simulink model "boost_fixed_irradiance"  (R2024b)
settings: Solver=ode5  StartTime=0.0  StopTime=5  MaxStep=1e-3  RelTol=1e-3
libraries: spsSeriesRLCBranchLib x3, spsCurrentMeasurementLib x1, spsDiodeLib x1, spsMosfetLib x1, slpidlib x1, spsPVArrayLib x1, spsPWMGeneratorDCDCLib x1, simulink x1, spsVoltageMeasurementLib x1, spspowerguiLib x1
settings Model: Creator=30698  LastModifiedBy=strat
settings SolverCC: AlgebraicLoopSolver=TrustRegion
settings DebuggingCC: UnconnectedInputMsg=warning  UnconnectedOutputMsg=warning  UnconnectedLineMsg=warning
settings ModelReferenceCC: EnableRefExpFcnMdlSchedulingChecks=on
settings RTWCC: GPUComputeCapability=3.5  DLArmComputeVersion=19.05

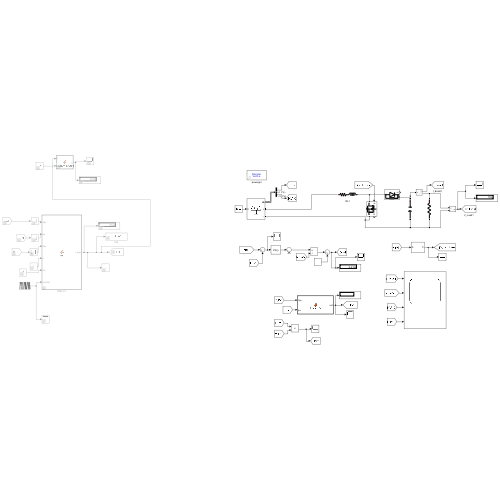
[thumbnail: Simulink's stored preview of the top-level diagram]
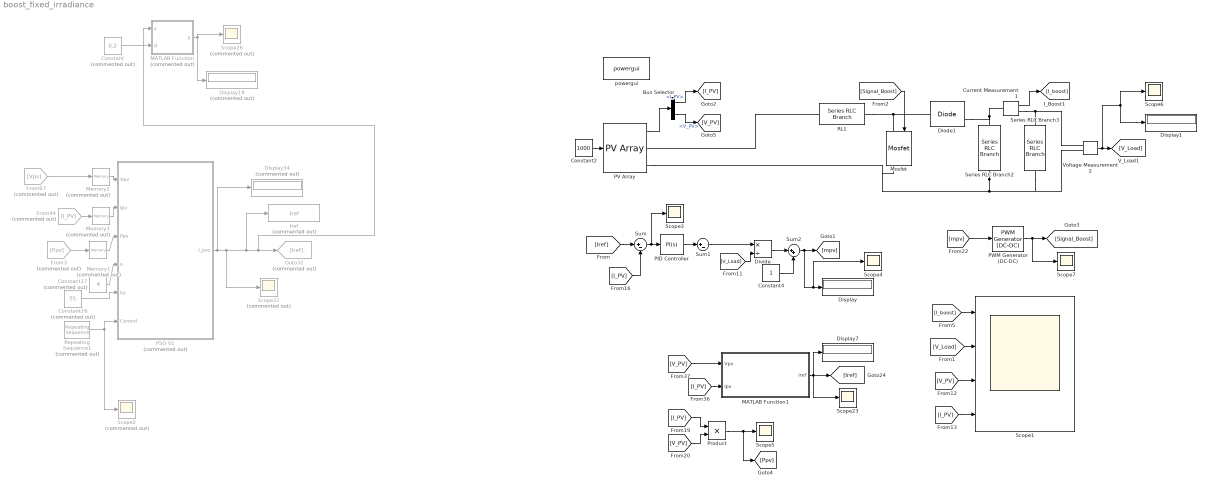
== system boost_fixed_irradiance ==
  Bus Selector : BusSelector  OutputSignals=I_PV,V_PV
  Constant : Constant  Commented=on  Value=0.2
  Constant16 : Constant  Commented=on  Value=55
  Constant17 : Constant  Commented=on  Value=4
  Constant2 : Constant  Value=1000
  Constant4 : Constant
  Current Measurement1 : spsCurrentMeasurementLib/Current Measurement  PhasorSimulation=off  OutputType=Complex  PSBequivalent=0
  Diode1 : spsDiodeLib/Diode  Ron=0.001  Lon=0  Vf=0.8  IC=0  UseSnubber=0  Rs=500  Cs=250e-9  Measurements=on
  Display : Display
  Display1 : Display
  Display19 : Display  Commented=on
  Display34 : Display  Commented=on
  Display7 : Display
  Divide : Product  Inputs=*/
  From3 : From  Commented=on  GotoTag=Ppv
  From44 : From  Commented=on  GotoTag=I_PV
  From67 : From  Commented=on  GotoTag=Vpv
  Goto32 : Goto  Commented=on  GotoTag=Iref
  Iref : ToWorkspace  Commented=on  VariableName=Iref  SaveFormat=Timeseries  SampleTime=-1
  MATLAB Function : MATLAB Function  Commented=on  TreatAsAtomicUnit=on
  MATLAB Function1 : MATLAB Function  TreatAsAtomicUnit=on
  Memory1 : Memory  Commented=on  InheritSampleTime=on
  Memory2 : Memory  Commented=on  InheritSampleTime=on
  Memory3 : Memory  Commented=on  InheritSampleTime=on
  Mosfet : spsMosfetLib/Mosfet  Ron=0.1  Lon=0  Rd=0.01  Vfd=0  IC=0  Rs=1e5  Cs=inf  Measurements=on
  PID Controller : slpidlib/PID Controller  Controller=PI  Form=Parallel  TimeDomain=Continuous-time  UseExternalTs=off  SampleTime=-1  IntegratorMethod=Forward Euler  FilterMethod=Forward Euler  ControllerParametersSource=internal  P=15  I=100  UseKiTs=off  D=0  UseExternalDerivativeSource=off  N=100  UseFilter=on  TunerSelectOption=Frequency Response Based  InitialConditionSource=internal  InitialConditionForIntegrator=0  InitialConditionForFilter=0  DifferentiatorICPrevScaledInput=0  ExternalReset=none  TrackingMode=off  Kt=1  LimitOutput=off  SatLimitsSource=internal  UpperSaturationLimit=inf  LowerSaturationLimit=-inf  LinearizeAsGain=on  AntiWindupMode=none  Kb=1  LimitIntegrator=off  UpperIntegratorSaturationLimit=inf  LowerIntegratorSaturationLimit=-inf  POutMin=[]  POutMax=[]  IOutMin=[]  IOutMax=[]  DOutMin=[]  DOutMax=[]  NOutMin=[]  NOutMax=[]  SumOutMin=[]  SumOutMax=[]  SaturationOutMin=[]  SaturationOutMax=[]  PParamMin=[]  PParamMax=[]  IParamMin=[]  IParamMax=[]  DParamMin=[]  DParamMax=[]  NParamMin=[]  NParamMax=[]  KbParamMin=[]  KbParamMax=[]  KtParamMin=[]  KtParamMax=[]  KbOutMin=[]  KbOutMax=[]  KtOutMin=[]  KtOutMax=[]  IntegratorOutMin=[]  IntegratorOutMax=[]  FilterOutMin=[]  FilterOutMax=[]  SumI1OutMin=[]  SumI1OutMax=[]  SumI2OutMin=[]  SumI2OutMax=[]  SumI3OutMin=[]  SumI3OutMax=[]  SumI4OutMin=[]  SumI4OutMax=[]  SumDOutMin=[]  SumDOutMax=[]  DifferentiatorOutMin=[]  DifferentiatorOutMax=[]  FilterDiffOutCoefMin=[]  FilterDiffOutCoefMax=[]  ReciprocalOutMin=[]  ReciprocalOutMax=[]  SumDenOutMin=[]  SumDenOutMax=[]  SumNumOutMin=[]  SumNumOutMax=[]  DivideOutMin=[]  DivideOutMax=[]  UdiffTsProdOutMin=[]  UdiffTsProdOutMax=[]  NTsProdOutMin=[]  NTsProdOutMax=[]  UintegralTsProdOutMin=[]  UintegralTsProdOutMax=[]  UngainTsProdOutMin=[]  UngainTsProdOutMax=[]  ClampingZeroOutDataTypeStr=Inherit: Inherit via back propagation  ClampingZeroOutMin=[]  ClampingZeroOutMax=[]  FilterDenConstantOutDataTypeStr=Inherit: Inherit via back propagation  FilterDenConstantOutMin=[]  FilterDenConstantOutMax=[]  PCopyOutDataTypeStr=Inherit: Inherit via back propagation  PCopyOutMin=[]  PCopyOutMax=[]  NCopyOutDataTypeStr=Inherit: Inherit via back propagation  NCopyOutMin=[]  NCopyOutMax=[]  IntegratorContinuousStateAttributes=''  IntegratorStateMustResolveToSignalObject=off  IntegratorRTWStateStorageClass=Auto  FilterContinuousStateAttributes=''  FilterStateMustResolveToSignalObject=off  FilterRTWStateStorageClass=Auto  ParallelPVariant=InternalParameters  IdealPVariant=Disabled  IVariant=InternalParameters  DVariant=Disabled  IntegratorVariant=Continuous  SatVariant=Disabled  AWVariant=Passthrough  PCopyVariant=Disabled  TRVariant=Disabled  FdbkBlocksVariant=Forward  IdealPFdbkVariant=Disabled  SatFdbkVariant=Disabled  DerivativeFilterVariant=Disabled  NVariant=Disabled  NCopyVariant=Disabled_SignalSpec  FilterICVariant=Disabled  IntegratorICVariant=InternalICs  ExternalResetVariant=Disabled  TRSumVariant=Passthrough  SumFdbkVariant=Disabled  SumVariant=Sum_PI  TsampFilterVariant=InternalTs  TsampNgainVariant=Passthrough  TsampIntegralVariant=Disabled_SignalSpec  ExternalSaturationOutDataTypeStr=Inherit: Same as second input  DerivativeSourceVariant=Disabled  PreIntVariant=InternalPreInt
  PSO V1 : MATLAB Function  Commented=on  TreatAsAtomicUnit=on  SystemSampleTime=1e-2
      settings: MinAlgLoopOccurrences=on
  PV Array : spsPVArrayLib/PV Array  Npar=5  Nser=14.15  PlotType=array @ 1000 W/m2 & specified temperatures  S_vec="[ 1000  500  100 ]"  Temp_C_vec="[ 45 25  ]"  ModuleName=User-defined  PlotWhenSelected=off  Pm=213.15  Ncell=60  Voc=34.7  Isc=7.84  Vm=29  Im=7.35  beta_Voc_pc=-0.36099  alpha_Isc_pc=0.102  beta_Voc=-0.12526  alpha_Isc=0.0079968  IL=7.8455  I0=2.9177e-10  nI=0.938  Rsh=259.7398  Rs=0.18261  RobustModel=on  RobustCellTemperature=25  BAL=on  Tc=1e-6  Tfilter=5e-5
  PWM Generator (DC-DC) : spsPWMGeneratorDCDCLib/PWM Generator (DC-DC)  Fsw=20000  Ts=0
  Product : Product
  RL1 : spsSeriesRLCBranchLib/Series RLC Branch  LConnTagsString=__new0  RConnTagsString=__new0  BranchType=RL  Resistance=0.01  Inductance=8e-3  SetiL0=off  InitialCurrent=0  Capacitance=1e-6  Setx0=off  InitialVoltage=0  Measurements=None
  Repeating Sequence1 : simulink/Sources/Repeating Sequence  Commented=on  rep_seq_t=[0 4.9 5 9 9.9 10 14]  rep_seq_y="[0 1 1 0  1 1 0]"
  Scope1 : Scope  NumInputPorts=4
  Scope2 : Scope  Commented=on
  Scope{3..7,23} (6 alike) : Scope
  Scope26 : Scope  Commented=on
  Scope31 : Scope  Commented=on
  Series RLC Branch2 : spsSeriesRLCBranchLib/Series RLC Branch  LConnTagsString=__new0  RConnTagsString=__new0  BranchType=C  Resistance=1  Inductance=1e-3  SetiL0=off  InitialCurrent=0  Capacitance=1e-2  Setx0=on  InitialVoltage=400  Measurements=None
  Series RLC Branch3 : spsSeriesRLCBranchLib/Series RLC Branch  LConnTagsString=__new0  RConnTagsString=__new0  BranchType=R  Resistance=100  Inductance=1e-3  SetiL0=off  InitialCurrent=0  Capacitance=1e-6  Setx0=off  InitialVoltage=0  Measurements=None
  Sum : Sum  Inputs=|+-
  Sum1 : Sum  Inputs=|+-
  Sum2 : Sum  Inputs=|++
  Voltage Measurement2 : spsVoltageMeasurementLib/Voltage Measurement  PhasorSimulation=off  OutputType=Complex  PSBequivalent=0
  powergui : spspowerguiLib/powergui  Priority=1  SimulationMode=Discrete  SampleTime=1e-5  frequency=60  Iterations=50  frequencyindice=0  Pbase=100e6  ErrMax=1e-4  UnitsV=kV  UnitsW=MW  buscounter=0  FunctionMessages=off  echomessages=off  EnableUseOfTLC=off  CurrentSourceSwitches=off  DisableSnubberDevices=off  DisableRonSwitches=off  DisableVfSwitches=off  DisplayEquations=off  AutomaticDiscreteSolvers=off  SolverType=Tustin/Backward Euler (TBE)  Interpol=off  ExternalGateDelay=off  methode=off  Ts=100  x0status=blocks  SPID=on  SwTol=0  HookPort=off  NonlinearTolerance=1e-4  nMaxIteration=100  ContinueOnMaxIteration=off  RestoreLinks=warning  ResistiveCurrentMeasurement=off  Frange=[0:2:500]  Ylog=off  Xlog=on  ShowGrid=off  save=off  variable=ZData  structure=0  ZoomFFT=off  StartTime=0.0  cycles=1  DisplayStyle=1  fundamental=60  FreqAxis=off  MaxFrequency=1000  frequencyindicesteady=1  RmsSteady=1  display=off
  wires:
  [I_boost] -> Scope1/1
  PWM Generator (DC-DC)/1 -> Scope7/1, [Signal_Boost]
  Bus Selector/2 -> [V_PV]  "<V_PV>"
  [V_Load] -> Scope1/2
  [V_PV] -> Scope1/3
  [I_PV] -> Scope1/4
  Sum/1 -> Scope3/1, PID Controller/1
  PID Controller/1 -> Sum1/1
  Sum1/1 -> Divide/1
  [V_Load] -> Divide/2
  Divide/1 -> Sum2/1
  Constant4/1 -> Sum2/2
  Sum2/1 -> [mpv], Scope4/1, Display/1
  [Iref] -> Sum/1
  [I_PV] -> Sum/2
  [I_PV] -> Product/1
  [V_PV] -> Product/2
  Product/1 -> [Ppv], Scope5/1
  Current Measurement1/1 -> [I_boost]
  [Signal_Boost] -> Mosfet/1
  Voltage Measurement2/1 -> Scope6/1, Display1/1, [V_Load]
  [mpv] -> PWM Generator (DC-DC)/1
  Bus Selector/1 -> [I_PV]  "<I_PV>"
  PV Array/1 -> Bus Selector/1
  [V_PV] -> MATLAB Function1/1(Vpv)
  [I_PV] -> MATLAB Function1/2(Ipv)
  MATLAB Function/1(y) -> Scope26/1, Display19/1
  MATLAB Function1/1(iref) -> Display7/1, [Iref], Scope23/1
  Constant/1 -> MATLAB Function/2(d)
  Memory3/1 -> PSO V1/2(Ipv)
  PSO V1/1(I_pso) -> MATLAB Function/1(x), Goto32/1, Iref/1, Scope31/1, Display34/1
  From3/1 -> Memory1/1
  Memory1/1 -> PSO V1/3(Ppv)
  Constant17/1 -> PSO V1/4(n)
  From67/1 -> Memory2/1
  From44/1 -> Memory3/1
  Constant16/1 -> PSO V1/5(Isc)
  Memory2/1 -> PSO V1/1(Vpv)
  Repeating Sequence1/1 -> PSO V1/6(Control), Scope2/1
  Constant2/1 -> PV Array/1
  connections:
  Series RLC Branch2/RConn1 -- PV Array/RConn2 -- Mosfet/RConn1 -- Series RLC Branch3/RConn1 -- Voltage Measurement2/LConn2
  RL1/RConn1 -- Diode1/LConn1 -- Mosfet/LConn1
  Series RLC Branch2/LConn1 -- Current Measurement1/LConn1 -- Diode1/RConn1
  Current Measurement1/RConn1 -- Series RLC Branch3/LConn1 -- Voltage Measurement2/LConn1
  RL1/LConn1 -- PV Array/RConn1

== matlab function boost_fixed_irradiance/MATLAB Function1 ==
  settings: updateMethod=DISCRETE
  data: Vpv input; Ipv input; iref output
function iref = P_and_O(Vpv, Ipv)
    persistent Vold Pold iref_old Ipv_old;
    if isempty(Vold) % Initialize Vold, Pold, and iref_old with isempty
        Vold = 0;
        Pold = 0;
        iref_old =0;
        Ipv_old=0;
    end
    P = Vpv * Ipv;
    dP = P - Pold;
    dVpv = Vpv - Vold;
    dI = Ipv - Ipv_old;
    d = 0.02;
    if dP ~= 0
        if dP > 0
            if dI > 0
                iref = iref_old + d; % Change iref directly inside the if loop
            else
                iref = iref_old - d;
            end
        else
            if dI > 0
                iref = iref_old - d; % Change iref directly inside the if loop
            else
                iref = iref_old + d;
            end
        end
    else
        iref = iref_old;
    end
    Vold = Vpv;
    Pold = P;
    iref_old = iref;
    Ipv_old=Ipv;
end

== matlab function boost_fixed_irradiance/MATLAB Function ==
  settings: updateMethod=DISCRETE
  data: x input; y output; d input
function y    = updateAndOutput(x,d)
    persistent prevInput;
    persistent tableData;
    % Initialize tableData as an empty array on the first call.
    if isempty(tableData)
        tableData = [];
    end
    % Check if the input is different from the previous input.
    if isempty(prevInput) 
        prevInput=0;
    end
    if x ~= prevInput && (x-prevInput>=d || x-prevInput<=-d)
        % Update the previous input with the current input.
        prevInput = x;

        % Add the current input value to the tableData.
        tableData = [tableData; x]
            % Output the current input value.
    end
    y = x;
end

== matlab function boost_fixed_irradiance/PSO V1 ==
  settings: updateMethod=DISCRETE
  data: Vpv input; I_pso output; Ipv input; Ppv input; n input; Isc input; Control input
function I_pso = PSO(Vpv,Ipv,Ppv,n,Isc,Control) 

persistent u;          % current particle
persistent Icurrent;   % current I
persistent p;          % power
persistent pbest;
persistent I;          % current
persistent v;          % velocity (delta I)
persistent counter;
persistent gbest;
if Control==1
    I_pso=37;
    counter = 0;
    Icurrent = 0.7*Isc;
    gbest = Icurrent;
    p = zeros(n,1);
    for j = 1:n
         p(j) = -100000000;
    end
    v = zeros(n,1);
    pbest = zeros(n,1);
    u = 0;
    I = zeros(n, 1);
    for j = 1:n
         I(j) = 15 + rand() * (Isc - 15);  % Generate a random value between 20 and Isc
    end
    return 
else

if isempty(counter)
    counter = 0;
end

if isempty(Icurrent)
    Icurrent = 0.7*Isc;
end

if isempty(gbest)
    gbest = Icurrent;
end

if isempty(p)
    p = zeros(n,1);
    for j = 1:n
         p(j) = -100000000;
    end
end

if isempty(v)
    v = zeros(n,1);
end

if isempty(pbest)
    pbest = zeros(n,1);
end

if isempty(u)
    u = 0;
end
if isempty(I)
    I = zeros(n, 1);
    for j = 1:n
         I(j) = 15 + rand() * (Isc - 15);  % Generate a random value between 20 and Isc
    end
end

% if (counter >= 1 && counter < 500)
%     I_pso = Icurrent;
%     counter = counter + 1;
%     return;
% end


counter = 0;

if (u >= 1 && u <= n)
    p(u)
    if ((Ppv) > p(u))
        p(u) = Ppv;
        pbest(u) = Icurrent
    end
end

u = u + 1;

if u == (n+2)
    u = 1;
end

if (u >= 1 && u <= n)
    I_pso = I(u);
    Icurrent = I_pso;
    counter = 1;
    return;
elseif u == (n+1)
    [m,i] = max(p);
    pbest
    gbest = pbest(i)
    I_pso = gbest;
    Icurrent = I_pso;
    counter = 1;
    for j = 1:n
        v(j) = updatevelocity(v(j), pbest(j), I(j), gbest);
        I(j) = updateI(I(j), v(j));
    end
    v
    I
    return
else
    I_pso = 30;
end
end
end



function vfinal = updatevelocity(vel, pobest, I, gwbest)

w = 0.9;
c1 = 1;
c2 = 1;

vfinal = w*vel + c1*(pobest-I) + c2*(gwbest-I);

end


function Ifinal = updateI(I, vel)

Ifinal = I + vel;

end
